simulink model "PV_module"  (Simulink 10.0)
settings: Solver=ode15s  StartTime=0.0  StopTime=25  MaxStep=0.4  RelTol=1e-3  EnableMultiTasking=on
libraries: elec_lib x36, nesl_utility x5, fl_lib x4, simulink x3
settings Model: Creator=Sanjay Lodwal  LastModifiedBy=bhisma
settings DataIOCC: LimitDataPoints=on
settings DebuggingCC: SolverPrmCheckMsg=warning  StateNameClashWarn=warning
settings GRTTargetCC: GeneratePreprocessorConditionals=Disable all  CombineOutputUpdateFcns=on  GRTInterface=off
settings ConfigComp: CovExternalEMLEnable=off
settings SimscapeCC: SimscapeNormalizeSystem=off

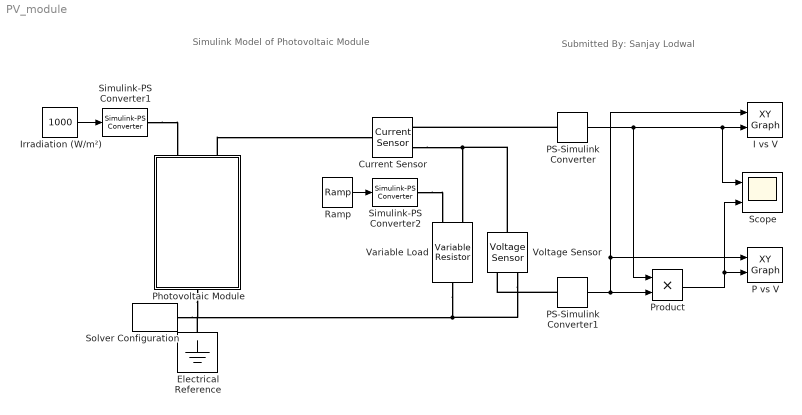
== system PV_module ==
  note: Simulink Model of Photovoltaic Module
  note: Submitted By: Sanjay Lodwal
  Current Sensor : fl_lib/Electrical/Electrical Sensors/Current Sensor  i1_Log=off  v1_Log=off  LocalVarNames=|i1|v1  LocalVarDescs=|i1|v1  LocalVarLogging=[0 0]
  Electrical Reference : fl_lib/Electrical/Electrical Elements/Electrical Reference  i_Log=off  LocalVarNames=|i  LocalVarDescs=|i  LocalVarLogging=0
  I vs V : simulink/Sinks/XY Graph  xmin=0  xmax=25  ymin=0  ymax=9  st=-1
  Irradiation (W/m²) : Constant  Value=1000
  P vs V : simulink/Sinks/XY Graph  xmin=0  xmax=25  ymin=0  ymax=165  st=-1
  PS-Simulink Converter : nesl_utility/PS-Simulink Converter  PhysicalDomain=network_engine_domain  SubClassName=ps_output  LeftPortType=input  RightPortType=output  PseudoPeriodic=off  Frequencies=[]  Unit=1  AffineConversion=off
  PS-Simulink Converter1 : nesl_utility/PS-Simulink Converter  PhysicalDomain=network_engine_domain  SubClassName=ps_output  LeftPortType=input  RightPortType=output  PseudoPeriodic=off  Frequencies=[]  Unit=1  AffineConversion=off
  Photovoltaic Module : Subsystem  mask{Voc=22.75, Isc=8.9, n=1.2, Rs=50e-3, Ir0=1000}
      mask prompts: Voc "Open circuit voltage"; Isc "Short circuit current"; n "Ideality factor"; Rs "Series resistance"; Ir0 "Reference irradiation"
      mask Display:
      | image('C:\Users\Sanjay Lodwal\Documents\MATLAB\Matlab_Final\pv_panel.jpg');
      | color('white');
  Product : Product
  Ramp : simulink/Sources/Ramp  slope=1  start=0  X0=0
  Scope : Scope  NumInputPorts=2
  Simulink-PS Converter1 : nesl_utility/Simulink-PS Converter  PhysicalDomain=network_engine_domain  SubClassName=ps_input  LeftPortType=input  RightPortType=output  PseudoPeriodic=off  Frequencies=[]  NoiseDistribution=none  NoiseParameters=[]  Unit=1  AffineConversion=off  InputFiltering=off  SimscapeFilterOrder=1  InputFilterTimeConstant=0.001  UdotUserProvided=1
  Simulink-PS Converter2 : nesl_utility/Simulink-PS Converter  PhysicalDomain=network_engine_domain  SubClassName=ps_input  LeftPortType=input  RightPortType=output  PseudoPeriodic=off  Frequencies=[]  NoiseDistribution=none  NoiseParameters=[]  Unit=1  AffineConversion=off  InputFiltering=off  SimscapeFilterOrder=1  InputFilterTimeConstant=0.001  UdotUserProvided=1
  Solver Configuration : nesl_utility/Solver Configuration  PhysicalDomain=network_engine_domain  SubClassName=solver  LeftPortType=input  RightPortType=generic  Accelerate=off  Tones=[]  Harmonics=[]  SimulateNoise=off  Profile=off  UseLocalSampling=off  EnableSwitchedLinearOptims=on  FrequencyDomain=off  UseCCode=off  UseNewInitialization=off  DoDC=off  ResidualTolerance=1e-09  UseLocalSolver=off  LocalSolverChoice=NE_BACKWARD_EULER_ADVANCER  LocalSolverSampleTime=0.001  DoFixedCost=off  MaxNonlinIter=3  MaxModeIter=2  LinearAlgebra=Sparse  DelaysMemoryBudget=1024
  Variable Load : fl_lib/Electrical/Electrical Elements/Variable Resistor  Rmin=0 Ohm  i_Log=off  v_Log=off  LocalVarNames=|i|v  LocalVarDescs=|i|v  LocalVarLogging=[0 0]
  Voltage Sensor : fl_lib/Electrical/Electrical Sensors/Voltage Sensor  i1_Log=off  v1_Log=off  LocalVarNames=|i1|v1  LocalVarDescs=|i1|v1  LocalVarLogging=[0 0]
  wires:
  Irradiation (W/m²)/1 -> Simulink-PS Converter1/1
  PS-Simulink Converter/1 -> I vs V/2, Scope/1, Product/1
  Product/1 -> P vs V/2, Scope/2
  Ramp/1 -> Simulink-PS Converter2/1
  PS-Simulink Converter1/1 -> Product/2, P vs V/1, I vs V/1
  connections:
  Simulink-PS Converter1/RConn1 -- Photovoltaic Module/RConn1
  Variable Load/RConn1 -- Voltage Sensor/RConn2 -- Photovoltaic Module/LConn1 -- Electrical Reference/LConn1 -- Solver Configuration/RConn1
  Simulink-PS Converter2/RConn1 -- Variable Load/LConn1
  Current Sensor/RConn2 -- Voltage Sensor/LConn1 -- Variable Load/LConn2
  Photovoltaic Module/RConn2 -- Current Sensor/LConn1
  PS-Simulink Converter/LConn1 -- Current Sensor/RConn1
  PS-Simulink Converter1/LConn1 -- Voltage Sensor/RConn1

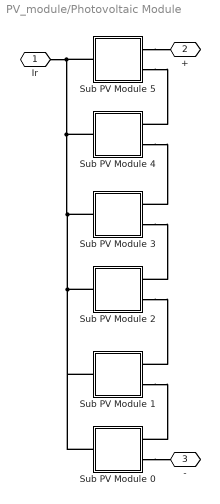
== system PV_module/Photovoltaic Module ==
  Sub PV Module 0 : Subsystem
  Sub PV Module 1 : Subsystem
  Sub PV Module 2 : Subsystem
  Sub PV Module 3 : Subsystem
  Sub PV Module 4 : Subsystem
  Sub PV Module 5 : Subsystem
  Ir : PMIOPort  Side=Right
  + : PMIOPort  Port=2  Side=Right
  - : PMIOPort  Port=3  Side=Left
  connections:
  Ir/RConn1 -- Sub PV Module 5/LConn1 -- Sub PV Module 4/LConn1 -- Sub PV Module 3/LConn1 -- Sub PV Module 2/LConn1 -- Sub PV Module 1/LConn1 -- Sub PV Module 0/LConn1
  Sub PV Module 3/RConn2 -- Sub PV Module 2/RConn1
  Sub PV Module 5/RConn1 -- +/RConn1
  Sub PV Module 0/RConn2 -- -/RConn1
  Sub PV Module 2/RConn2 -- Sub PV Module 1/RConn1
  Sub PV Module 1/RConn2 -- Sub PV Module 0/RConn1
  Sub PV Module 5/RConn2 -- Sub PV Module 4/RConn1
  Sub PV Module 4/RConn2 -- Sub PV Module 3/RConn1

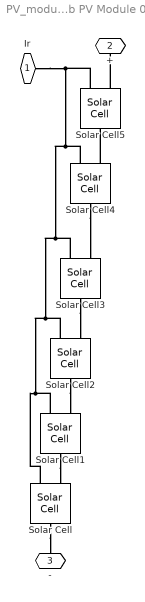
== system PV_module/Photovoltaic Module/Sub PV Module 0 ==
  Solar Cell{,1..5} (6 alike) : elec_lib/Sources/Solar Cell  prm=1  Isc=Isc A  Voc=Voc/36 V  Is=1e-6 A  Is2=0 A  Iph=7.34 A  Ir0=Ir0 W/m^2  ec=n  N2=2  Rs=Rs/36 Ohm  Rp=Inf Ohm  TIPH1=0 1/K  EG=1.11 eV  TXIS1=3  TXIS2=3  TRS1=0  TRP1=0  Tmeas=25 C  TFIXED=25 C  LocalVarLogging=[]  thermal_mass=100 J/K  initial_temperature=25 C
      settings: SourceProductName=Simscape Electrical  SourceProductBaseCode=PS
  Ir : PMIOPort  Side=Left
  + : PMIOPort  Port=2  Side=Right
  - : PMIOPort  Port=3  Side=Right
  connections:
  Solar Cell1/RConn1 -- Solar Cell/LConn2
  Solar Cell4/RConn1 -- Solar Cell3/LConn2
  Solar Cell3/RConn1 -- Solar Cell2/LConn2
  Solar Cell2/RConn1 -- Solar Cell1/LConn2
  Solar Cell/RConn1 -- -/RConn1
  Solar Cell5/LConn2 -- +/RConn1
  Solar Cell4/LConn1 -- Solar Cell5/LConn1 -- Ir/RConn1 -- Solar Cell3/LConn1 -- Solar Cell2/LConn1 -- Solar Cell1/LConn1 -- Solar Cell/LConn1
  Solar Cell4/LConn2 -- Solar Cell5/RConn1

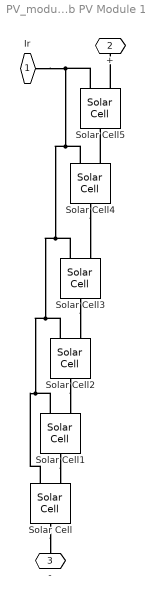
== system PV_module/Photovoltaic Module/Sub PV Module 1 ==
  Solar Cell{,1..5} (6 alike) : elec_lib/Sources/Solar Cell  prm=1  Isc=Isc A  Voc=Voc/36 V  Is=1e-6 A  Is2=0 A  Iph=7.34 A  Ir0=Ir0 W/m^2  ec=n  N2=2  Rs=Rs/36 Ohm  Rp=Inf Ohm  TIPH1=0 1/K  EG=1.11 eV  TXIS1=3  TXIS2=3  TRS1=0  TRP1=0  Tmeas=25 C  TFIXED=25 C  LocalVarLogging=[]  thermal_mass=100 J/K  initial_temperature=25 C
      settings: SourceProductName=Simscape Electrical  SourceProductBaseCode=PS
  Ir : PMIOPort  Side=Left
  + : PMIOPort  Port=2  Side=Right
  - : PMIOPort  Port=3  Side=Right
  connections:
  Solar Cell1/RConn1 -- Solar Cell/LConn2
  Solar Cell4/RConn1 -- Solar Cell3/LConn2
  Solar Cell3/RConn1 -- Solar Cell2/LConn2
  Solar Cell2/RConn1 -- Solar Cell1/LConn2
  Solar Cell/RConn1 -- -/RConn1
  Solar Cell5/LConn2 -- +/RConn1
  Solar Cell3/LConn1 -- Solar Cell2/LConn1 -- Solar Cell1/LConn1 -- Solar Cell/LConn1 -- Solar Cell5/LConn1 -- Ir/RConn1 -- Solar Cell4/LConn1
  Solar Cell4/LConn2 -- Solar Cell5/RConn1

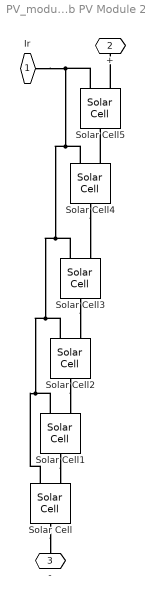
== system PV_module/Photovoltaic Module/Sub PV Module 2 ==
  Solar Cell{,1..5} (6 alike) : elec_lib/Sources/Solar Cell  prm=1  Isc=Isc A  Voc=Voc/36 V  Is=1e-6 A  Is2=0 A  Iph=7.34 A  Ir0=Ir0 W/m^2  ec=n  N2=2  Rs=Rs/36 Ohm  Rp=Inf Ohm  TIPH1=0 1/K  EG=1.11 eV  TXIS1=3  TXIS2=3  TRS1=0  TRP1=0  Tmeas=25 C  TFIXED=25 C  LocalVarLogging=[]  thermal_mass=100 J/K  initial_temperature=25 C
      settings: SourceProductName=Simscape Electrical  SourceProductBaseCode=PS
  Ir : PMIOPort  Side=Left
  + : PMIOPort  Port=2  Side=Right
  - : PMIOPort  Port=3  Side=Right
  connections:
  Solar Cell1/RConn1 -- Solar Cell/LConn2
  Solar Cell4/RConn1 -- Solar Cell3/LConn2
  Solar Cell3/RConn1 -- Solar Cell2/LConn2
  Solar Cell2/RConn1 -- Solar Cell1/LConn2
  Solar Cell/RConn1 -- -/RConn1
  Solar Cell5/LConn2 -- +/RConn1
  Solar Cell3/LConn1 -- Solar Cell2/LConn1 -- Solar Cell1/LConn1 -- Solar Cell/LConn1 -- Solar Cell5/LConn1 -- Ir/RConn1 -- Solar Cell4/LConn1
  Solar Cell4/LConn2 -- Solar Cell5/RConn1

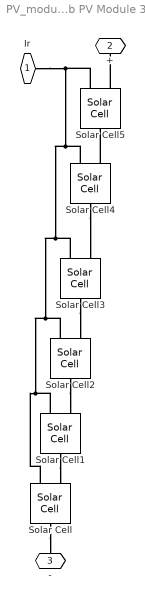
== system PV_module/Photovoltaic Module/Sub PV Module 3 ==
  Solar Cell{,1..5} (6 alike) : elec_lib/Sources/Solar Cell  prm=1  Isc=Isc A  Voc=Voc/36 V  Is=1e-6 A  Is2=0 A  Iph=7.34 A  Ir0=Ir0 W/m^2  ec=n  N2=2  Rs=Rs/36 Ohm  Rp=Inf Ohm  TIPH1=0 1/K  EG=1.11 eV  TXIS1=3  TXIS2=3  TRS1=0  TRP1=0  Tmeas=25 C  TFIXED=25 C  LocalVarLogging=[]  thermal_mass=100 J/K  initial_temperature=25 C
      settings: SourceProductName=Simscape Electrical  SourceProductBaseCode=PS
  Ir : PMIOPort  Side=Left
  + : PMIOPort  Port=2  Side=Right
  - : PMIOPort  Port=3  Side=Right
  connections:
  Solar Cell1/RConn1 -- Solar Cell/LConn2
  Solar Cell4/RConn1 -- Solar Cell3/LConn2
  Solar Cell3/RConn1 -- Solar Cell2/LConn2
  Solar Cell2/RConn1 -- Solar Cell1/LConn2
  Solar Cell/RConn1 -- -/RConn1
  Solar Cell5/LConn2 -- +/RConn1
  Solar Cell3/LConn1 -- Solar Cell2/LConn1 -- Solar Cell1/LConn1 -- Solar Cell/LConn1 -- Solar Cell5/LConn1 -- Ir/RConn1 -- Solar Cell4/LConn1
  Solar Cell4/LConn2 -- Solar Cell5/RConn1

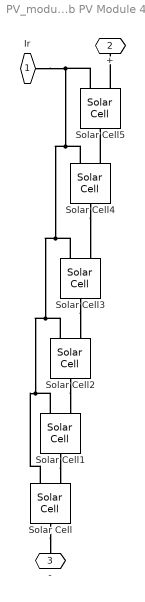
== system PV_module/Photovoltaic Module/Sub PV Module 4 ==
  Solar Cell{,1..5} (6 alike) : elec_lib/Sources/Solar Cell  prm=1  Isc=Isc A  Voc=Voc/36 V  Is=1e-6 A  Is2=0 A  Iph=7.34 A  Ir0=Ir0 W/m^2  ec=n  N2=2  Rs=Rs/36 Ohm  Rp=Inf Ohm  TIPH1=0 1/K  EG=1.11 eV  TXIS1=3  TXIS2=3  TRS1=0  TRP1=0  Tmeas=25 C  TFIXED=25 C  LocalVarLogging=[]  thermal_mass=100 J/K  initial_temperature=25 C
      settings: SourceProductName=Simscape Electrical  SourceProductBaseCode=PS
  Ir : PMIOPort  Side=Left
  + : PMIOPort  Port=2  Side=Right
  - : PMIOPort  Port=3  Side=Right
  connections:
  Solar Cell1/RConn1 -- Solar Cell/LConn2
  Solar Cell4/RConn1 -- Solar Cell3/LConn2
  Solar Cell3/RConn1 -- Solar Cell2/LConn2
  Solar Cell2/RConn1 -- Solar Cell1/LConn2
  Solar Cell/RConn1 -- -/RConn1
  Solar Cell5/LConn2 -- +/RConn1
  Solar Cell3/LConn1 -- Solar Cell2/LConn1 -- Solar Cell1/LConn1 -- Solar Cell/LConn1 -- Solar Cell5/LConn1 -- Ir/RConn1 -- Solar Cell4/LConn1
  Solar Cell4/LConn2 -- Solar Cell5/RConn1

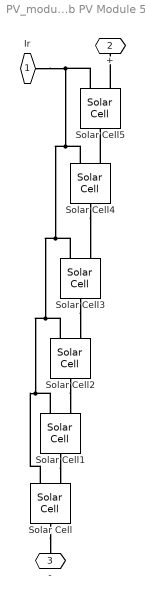
== system PV_module/Photovoltaic Module/Sub PV Module 5 ==
  Solar Cell{,1..5} (6 alike) : elec_lib/Sources/Solar Cell  prm=1  Isc=Isc A  Voc=Voc/36 V  Is=1e-6 A  Is2=0 A  Iph=7.34 A  Ir0=Ir0 W/m^2  ec=n  N2=2  Rs=Rs/36 Ohm  Rp=Inf Ohm  TIPH1=0 1/K  EG=1.11 eV  TXIS1=3  TXIS2=3  TRS1=0  TRP1=0  Tmeas=25 C  TFIXED=25 C  LocalVarLogging=[]  thermal_mass=100 J/K  initial_temperature=25 C
      settings: SourceProductName=Simscape Electrical  SourceProductBaseCode=PS
  Ir : PMIOPort  Side=Left
  + : PMIOPort  Port=2  Side=Right
  - : PMIOPort  Port=3  Side=Right
  connections:
  Solar Cell1/RConn1 -- Solar Cell/LConn2
  Solar Cell4/RConn1 -- Solar Cell3/LConn2
  Solar Cell3/RConn1 -- Solar Cell2/LConn2
  Solar Cell2/RConn1 -- Solar Cell1/LConn2
  Solar Cell/RConn1 -- -/RConn1
  Solar Cell5/LConn2 -- +/RConn1
  Solar Cell3/LConn1 -- Solar Cell2/LConn1 -- Solar Cell1/LConn1 -- Solar Cell/LConn1 -- Solar Cell5/LConn1 -- Ir/RConn1 -- Solar Cell4/LConn1
  Solar Cell4/LConn2 -- Solar Cell5/RConn1
